simulink model "Graph1"  (R2017b)
settings: Solver=VariableStepAuto  StartTime=0.0  StopTime=10  RelTol=1e-3
values from neighbouring files (symbols this model uses):
  CD = -2    [Constants1.m]    (also in Tank.m; tankproblem.m)
  gc = -32.2    [Constants1.m]    (also in Tank.m; tankproblem.m)
  m = -3.1677018633540368    (= -3.16770186335)    [Constants1.m]    (also in Tank.m; tankproblem.m)
settings Model: Creator=justi  LastModifiedBy=justi

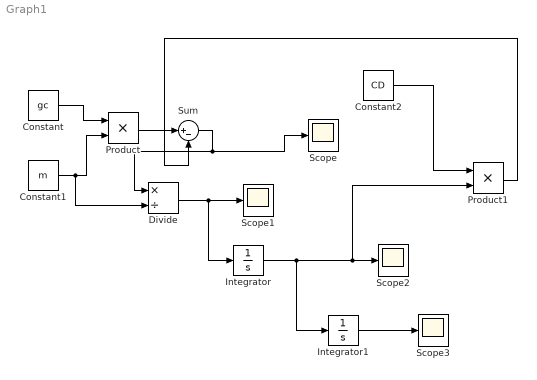
== system Graph1 ==
  Constant : Constant  Value=gc
  Constant1 : Constant  Value=m
  Constant2 : Constant  Value=CD
  Divide : Product  Inputs=*/
  Integrator : Integrator  InitialCondition=200
  Integrator1 : Integrator  InitialCondition=10
  Product : Product
  Product1 : Product
  Scope{,1..3} (4 alike) : Scope
  Sum : Sum  Inputs=|+-
  wires:
  Constant/1 -> Product/1
  Constant1/1 -> Divide/2, Product/2
  Product/1 -> Sum/1
  Sum/1 -> Divide/1, Scope/1
  Divide/1 -> Integrator/1, Scope1/1
  Product1/1 -> Sum/2
  Constant2/1 -> Product1/1
  Integrator1/1 -> Scope3/1
  Integrator/1 -> Integrator1/1, Product1/2, Scope2/1
